simulink model "lecture8_alarm"  (Simulink 7.1)
settings: Solver=FixedStepDiscrete  StartTime=0.0  StopTime=Inf  RelTol=1e-3
libraries: simulink x4
settings Model: Creator=pit  LastModifiedBy=pit

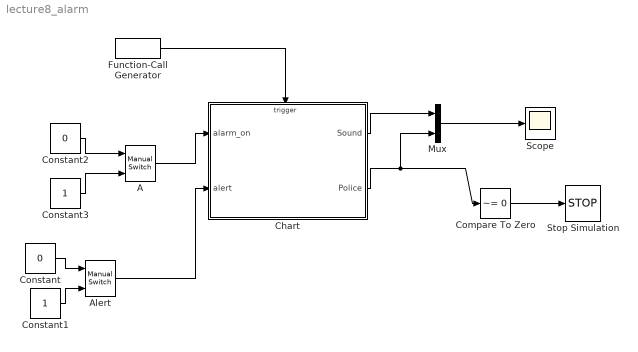
== system lecture8_alarm ==
  A : simulink/Signal Routing/Manual Switch  SystemSampleTime=-1  sw=1  action=0  varsize=off
  Alert : simulink/Signal Routing/Manual Switch  SystemSampleTime=-1  sw=0  action=0  varsize=off
  Chart : Stateflow chart
  Compare To Zero : simulink/Logic and Bit Operations/Compare To Zero  SystemSampleTime=-1  relop=~=  LogicOutDataTypeMode=boolean  ZeroCross=off
  Constant : Constant  Value=0  OutDataType=sfix(16)  OutScaling=2^0
  Constant1 : Constant  OutDataType=sfix(16)  OutScaling=2^0
  Constant2 : Constant  Value=0  OutDataType=sfix(16)  OutScaling=2^0
  Constant3 : Constant  OutDataType=sfix(16)  OutScaling=2^0
  Function-Call Generator : simulink/Ports & Subsystems/Function-Call Generator  sample_time=.05  numberOfIterations=1
  Mux : Mux  Inputs=2
  Scope : Scope
  Stop Simulation : Stop
  wires:
  Mux/1 -> Scope/1
  Chart/1(Sound) -> Mux/1
  Chart/2(Police) -> Mux/2, Compare To Zero/1
  Compare To Zero/1 -> Stop Simulation/1
  Constant2/1 -> A/1
  Constant3/1 -> A/2
  A/1 -> Chart/1(alarm_on)
  Function-Call Generator/1 -> Chart/Trigger
  Alert/1 -> Chart/2(alert)
  Constant/1 -> Alert/1
  Constant1/1 -> Alert/2

== stateflow chart Chart ==
  state On
    on Warn: Sound
    state Idle
    state Pending
      entry: Warn
    Pending -> Idle : after(10000,sec)/Police
    Idle -> Pending : [alert==1]
    (default) -> Idle
  state Off
  On -> Off : [alarm_on==0]
  Off -> On : [alarm_on==1]
  (default) -> On
  data: alarm_on input double; alert input double
  events: Sound output EITHER_EDGE_EVENT; Police output EITHER_EDGE_EVENT; Warn local EITHER_EDGE_EVENT; sl_call input FUNCTION_CALL_EVENT
